simulink model "verify_Flow_Mixer_basic_mdl"  (R2013b)
settings: Solver=VariableStepDiscrete  StartTime=0.0  StopTime=10.0  MaxStep=0.1  RelTol=1e-3
libraries: carnot x5
settings Model: Creator=drhf  LastModifiedBy=drhf
settings OptimizationCC: ExpressionDepthLimit=2147483647
settings DebuggingCC: StateNameClashWarn=warning
settings GRTTargetCC: CombineOutputUpdateFcns=off  GRTInterface=on

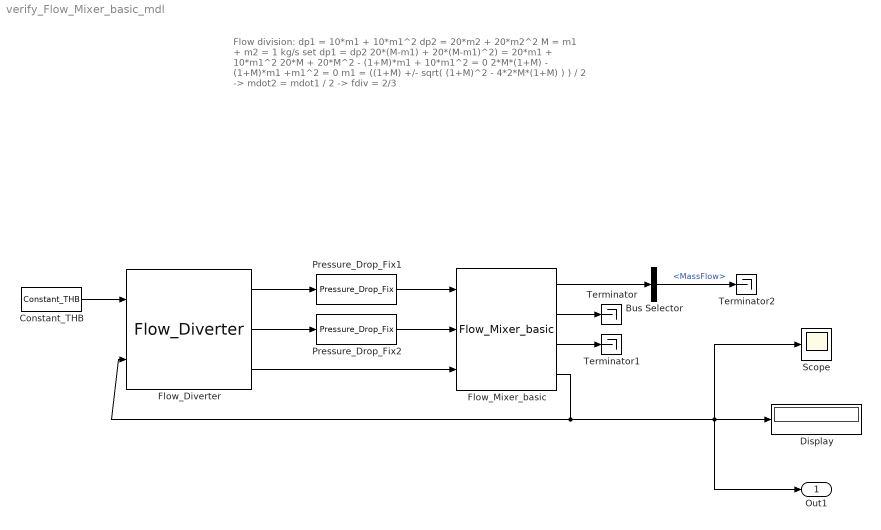
== system verify_Flow_Mixer_basic_mdl ==
  note: Flow division:
      | dp1 = 10*m1 + 10*m1^2
      | dp2 = 20*m2 + 20*m2^2
      | M = m1 + m2 = 1 kg/s
      | set dp1 = dp2
      | 20*(M-m1) + 20*(M-m1)^2) = 20*m1 + 10*m1^2
      | 20*M + 20*M^2 - (1+M)*m1 + 10*m1^2 = 0
      | 2*M*(1+M) - (1+M)*m1 +m1^2 = 0
      | m1 = ((1+M) +/- sqrt( (1+M)^2 - 4*2*M*(1+M) ) ) / 2
      |
      | -> mdot2 = mdot1 / 2
      | -> fdiv = 2/3
  Bus Selector : BusSelector  OutputSignals=MassFlow
  Constant_THB : carnot/Source/Simple/Constant_THB  t=40  mdot=1  p=1e5  mID=No Pressure Drop  fluid=Water  mix=0  mix2=0  mix3=0  dia=0.1  hgt=0
  Display : Display
  Flow_Diverter : carnot/Hydraulics/Flow_Diverter
  Flow_Mixer_basic : carnot/Basic/Hydraulics/Flow_Mixer_basic
  Pressure_Drop_Fix1 : carnot/Basic/Pressure_Drop/Pressure_Drop_Fix  con=0  lin=10  qua=0
  Pressure_Drop_Fix2 : carnot/Basic/Pressure_Drop/Pressure_Drop_Fix  con=0  lin=20  qua=0
  Scope : Scope
  Terminator : Terminator
  Terminator1 : Terminator
  Terminator2 : Terminator
  Out1 : Outport
  wires:
  Flow_Mixer_basic/4 -> Scope/1, Out1/1, Display/1, Flow_Diverter/2
  Flow_Diverter/1 -> Pressure_Drop_Fix1/1
  Flow_Diverter/2 -> Pressure_Drop_Fix2/1
  Constant_THB/1 -> Flow_Diverter/1
  Flow_Diverter/3 -> Flow_Mixer_basic/3
  Flow_Mixer_basic/2 -> Terminator/1
  Flow_Mixer_basic/3 -> Terminator1/1
  Pressure_Drop_Fix1/1 -> Flow_Mixer_basic/1
  Pressure_Drop_Fix2/1 -> Flow_Mixer_basic/2
  Flow_Mixer_basic/1 -> Bus Selector/1
  Bus Selector/1 -> Terminator2/1  "<MassFlow>"
